simulink model "Two_Level_Inverter"  (R2016a)
settings: Solver=VariableStepAuto  StartTime=0.0  StopTime=0.3  RelTol=1e-3
libraries: powerlib x10, simulink x1
settings Model: Creator=shahinSabour  LastModifiedBy=shahin

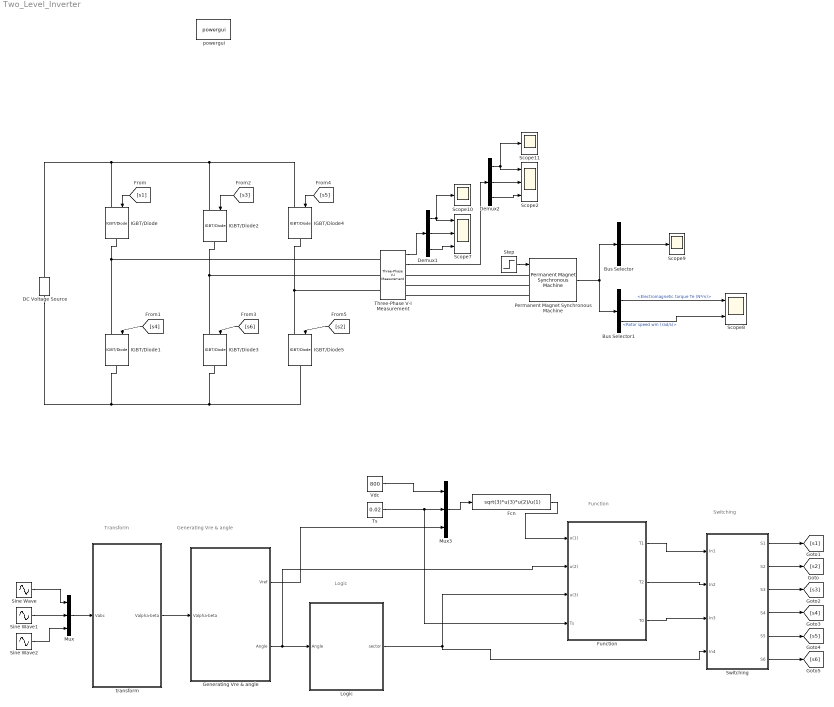
== system Two_Level_Inverter ==
  note: Transform
  note: Generating Vre & angle
  note: Logic
  note: Function
  note: Switching
  " transform" : Subsystem
  Bus Selector : BusSelector  OutputSignals=Stator current is_a (A),Stator current is_b (A),Stator current is_c (A)  OutputAsBus=on
  Bus Selector1 : BusSelector  OutputSignals=Electromagnetic torque Te (N*m),Rotor speed wm (rad/s)
  DC Voltage Source : powerlib/Electrical Sources/DC Voltage Source  Amplitude=800  Measurements=None
  Demux1 : Demux  Outputs=3
  Demux2 : Demux  Outputs=3
  Fcn : Fcn  Expr=sqrt(3)*u(3)*u(2)/u(1)
  Function : Subsystem
  Generating Vre & angle : Subsystem
  IGBT/Diode{,1..5} (6 alike) : powerlib/Power Electronics/IGBT//Diode  Ron=1e-3  Rs=1e5  Cs=inf  Measurements=off
  Logic : Subsystem
  Mux : Mux  Inputs=3
  Mux3 : Mux  Inputs=3
  Permanent Magnet Synchronous Machine : powerlib/Machines/Permanent Magnet Synchronous Machine  NbPhases=3  FluxDistribution=Sinusoidal  RotorType=Round  MechanicalLoad=Torque Tm  PresetModel="03:  2.8 Nm 300 Vdc 4250 RPM - 3.2 Nm"  ShowDetailedParameters=on  MeasurementBus=off  Resistance=1.6  Inductance=8.5e-3  dqInductances=[8.5e-3,8.5e-3]  La=0.006365  MachineConstant=Flux linkage established by magnets (V.s)  Flux=0.1852  VoltageCst=67.1831  TorqueCst=0.5556  Flat=120  Mechanical=[0.0001854 5.396e-05 2 0]  PolePairs=2  InitialConditions=[0,0, 0,0]  InitialConditions5ph=[0 0 0 0 0 0]  TsPowergui=0  TsBlock=-1  RefAngle=90 degrees behind phase A axis (modified Park)
  Scope10 : Scope
  Scope11 : Scope
  Scope2 : Scope  NumInputPorts=3
  Scope7 : Scope  NumInputPorts=3
  Scope8 : Scope  NumInputPorts=2
  Scope9 : Scope
  Sine Wave : Sin  Amplitude=800  Frequency=2*pi*50  SampleTime=0
  Sine Wave1 : Sin  Amplitude=800  Frequency=2*pi*50  Phase=2*pi/3  SampleTime=0
  Sine Wave2 : Sin  Amplitude=800  Frequency=2*pi*50  Phase=-2*pi/3  SampleTime=0
  Step : Step  Time=0.8  After=3  SampleTime=0
  "Switching " : Subsystem
  Three-Phase V-I Measurement : powerlib/Measurements/Three-Phase V-I Measurement  VoltageMeasurement=phase-to-phase  SetLabelV=off  LabelV=Vabc  Vpu=off  VpuLL=off  CurrentMeasurement=yes  SetLabelI=off  LabelI=Iabc  Ipu=off  Pbase=100e6  Vbase=500e3  OutputType=Complex  PhasorSimulation=off  PSBequivalent=0
  Ts : Constant  Value=0.02
  Vdc : Constant  Value=800
  powergui : powerlib/powergui  Priority=1  SimulationMode=Discrete  SolverType=Tustin/Backward Euler (TBE)  SampleTime=1e-7  frequency=60  SPID=off  DisableSnubberDevices=off  DisableRonSwitches=off  DisableVfSwitches=off  SwTol=0  DisplayEquations=off  Interpol=off  ExternalGateDelay=off  methode=off  Ts=10  FunctionMessages=off  echomessages=off  HookPort=off  EnableUseOfTLC=off  x0status=blocks  frequencyindice=0  Pbase=100e6  ErrMax=1e-4  Iterations=50  UnitsV=kV  UnitsW=MW  buscounter=0  RestoreLinks=warning  ResistiveCurrentMeasurement=off  Frange=[0:2:500]  Ylog=off  Xlog=on  ShowGrid=off  save=off  variable=ZData  structure=i  ZoomFFT=off  StartTime=0.2  cycles=1  DisplayStyle=1  fundamental=50  FreqAxis=on  MaxFrequency=1000  frequencyindicesteady=1  RmsSteady=1  display=off
  wires:
  Sine Wave/1 -> Mux/1
  Sine Wave1/1 -> Mux/2
  Sine Wave2/1 -> Mux/3
  Mux/1 -> " transform"/1(Vabc)
  " transform"/1(Valpha-beta) -> Generating Vre & angle/1(Valpha-beta)
  Generating Vre & angle/2(Angle) -> Function/2(u(2)), Logic/1(Angle)
  Generating Vre & angle/1(Vref) -> Mux3/3
  Ts/1 -> Function/4(Ts), Mux3/2
  Vdc/1 -> Mux3/1
  Mux3/1 -> Fcn/1
  Fcn/1 -> Function/1(u(1))
  Logic/1(sector) -> "Switching "/4(In4), Function/3(u(3))
  Permanent Magnet Synchronous Machine/1 -> Bus Selector1/1, Bus Selector/1
  Bus Selector1/1 -> Scope8/1  "<Electromagnetic torque Te (N*m)>"
  Bus Selector1/2 -> Scope8/2  "<Rotor speed wm (rad/s)>"
  Bus Selector/1 -> Scope9/1
  Step/1 -> Permanent Magnet Synchronous Machine/1
  Three-Phase V-I Measurement/1 -> Demux1/1
  Demux1/1 -> Scope10/1, Scope7/1
  Demux1/2 -> Scope7/2
  Demux1/3 -> Scope7/3
  Three-Phase V-I Measurement/2 -> Demux2/1
  Demux2/1 -> Scope2/1, Scope11/1
  Demux2/2 -> Scope2/2
  Demux2/3 -> Scope2/3
  [s5] -> IGBT/Diode4/1
  [s3] -> IGBT/Diode2/1
  [s6] -> IGBT/Diode3/1
  [s2] -> IGBT/Diode5/1
  [s4] -> IGBT/Diode1/1
  [s1] -> IGBT/Diode/1
  Function/1(T1) -> "Switching "/1(In1)
  Function/2(T2) -> "Switching "/2(In2)
  Function/3(T0) -> "Switching "/3(In3)
  "Switching "/2(S2) -> [s2]
  "Switching "/1(S1) -> [s1]
  "Switching "/3(S3) -> [s3]
  "Switching "/4(S4) -> [s4]
  "Switching "/5(S5) -> [s5]
  "Switching "/6(S6) -> [s6]
  connections:
  Permanent Magnet Synchronous Machine/LConn1 -- Three-Phase V-I Measurement/RConn1
  Permanent Magnet Synchronous Machine/LConn2 -- Three-Phase V-I Measurement/RConn2
  Permanent Magnet Synchronous Machine/LConn3 -- Three-Phase V-I Measurement/RConn3
  IGBT/Diode1/RConn1 -- DC Voltage Source/LConn1 -- IGBT/Diode3/RConn1 -- IGBT/Diode5/RConn1
  IGBT/Diode/RConn1 -- Three-Phase V-I Measurement/LConn1 -- IGBT/Diode1/LConn1
  IGBT/Diode/LConn1 -- DC Voltage Source/RConn1 -- IGBT/Diode2/LConn1 -- IGBT/Diode4/LConn1
  IGBT/Diode4/RConn1 -- Three-Phase V-I Measurement/LConn3 -- IGBT/Diode5/LConn1
  IGBT/Diode2/RConn1 -- Three-Phase V-I Measurement/LConn2 -- IGBT/Diode3/LConn1

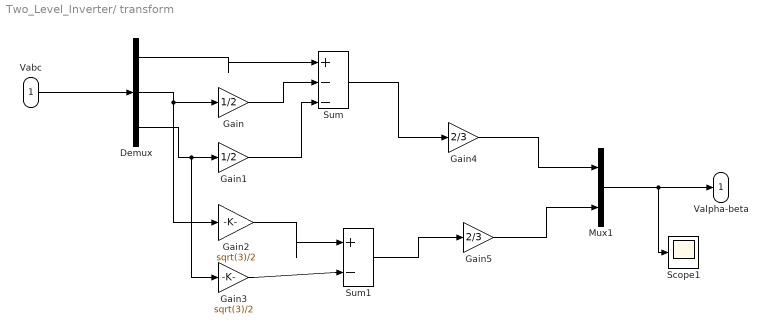
== system Two_Level_Inverter/ transform ==
  Vabc : Inport
  Demux : Demux  Outputs=3
  Gain : Gain  Gain=1/2
  Gain1 : Gain  Gain=1/2
  Gain2 : Gain  Gain=sqrt(3)/2
  Gain3 : Gain  Gain=sqrt(3)/2
  Gain4 : Gain  Gain=2/3
  Gain5 : Gain  Gain=2/3
  Mux1 : Mux  Inputs=2
  Scope1 : Scope
  Sum : Sum  Inputs=|+--
  Sum1 : Sum  Inputs=|+-
  Valpha-beta : Outport
  wires:
  Gain2/1 -> Sum1/1
  Gain5/1 -> Mux1/2
  Demux/3 -> Gain3/1, Gain1/1
  Demux/1 -> Sum/1
  Gain1/1 -> Sum/3
  Gain3/1 -> Sum1/2
  Demux/2 -> Gain2/1, Gain/1
  Mux1/1 -> Valpha-beta/1, Scope1/1
  Sum/1 -> Gain4/1
  Gain/1 -> Sum/2
  Sum1/1 -> Gain5/1
  Gain4/1 -> Mux1/1
  Vabc/1 -> Demux/1

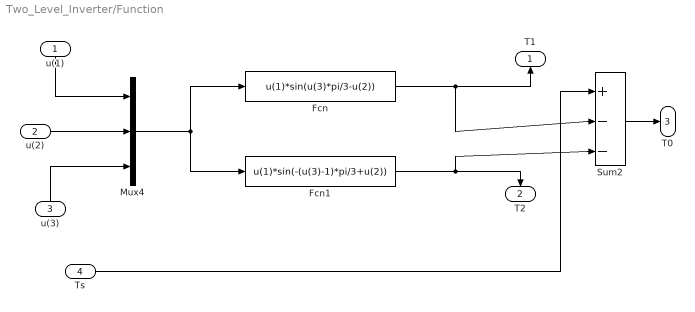
== system Two_Level_Inverter/Function ==
  u(1) : Inport
  u(2) : Inport  Port=2
  u(3) : Inport  Port=3
  Ts : Inport  Port=4
  Fcn : Fcn  Expr=u(1)*sin(u(3)*pi/3-u(2))
  Fcn1 : Fcn  Expr=u(1)*sin(-(u(3)-1)*pi/3+u(2))
  Mux4 : Mux  Inputs=3
  Sum2 : Sum  Inputs=|+--
  T1 : Outport
  T2 : Outport  Port=2
  T0 : Outport  Port=3
  wires:
  u(3)/1 -> Mux4/3
  u(2)/1 -> Mux4/2
  u(1)/1 -> Mux4/1
  Sum2/1 -> T0/1
  Fcn/1 -> Sum2/2, T1/1
  Ts/1 -> Sum2/1
  Fcn1/1 -> T2/1, Sum2/3
  Mux4/1 -> Fcn1/1, Fcn/1

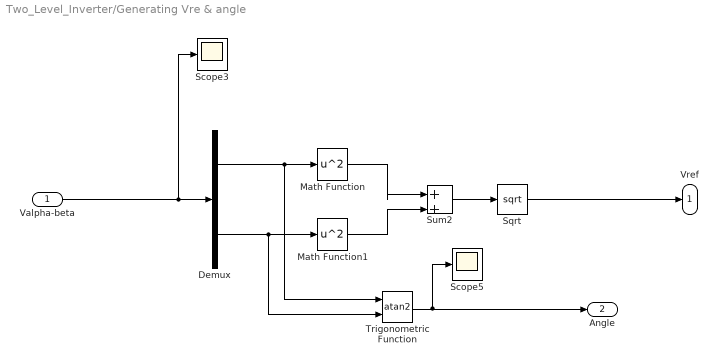
== system Two_Level_Inverter/Generating Vre & angle ==
  Valpha-beta : Inport
  Demux : Demux  Outputs=2
  Math Function : Math  Operator=square  SaturateOnIntegerOverflow=on
  Math Function1 : Math  Operator=square  SaturateOnIntegerOverflow=on
  Scope3 : Scope
  Scope5 : Scope
  Sqrt : Sqrt  SaturateOnIntegerOverflow=on
  Sum2 : Sum  Inputs=|++
  Trigonometric Function : Trigonometry  Operator=atan2
  Vref : Outport
  Angle : Outport  Port=2
  wires:
  Valpha-beta/1 -> Scope3/1, Demux/1
  Sqrt/1 -> Vref/1
  Math Function/1 -> Sum2/1
  Math Function1/1 -> Sum2/2
  Demux/2 -> Trigonometric Function/2, Math Function1/1
  Demux/1 -> Trigonometric Function/1, Math Function/1
  Sum2/1 -> Sqrt/1
  Trigonometric Function/1 -> Angle/1, Scope5/1

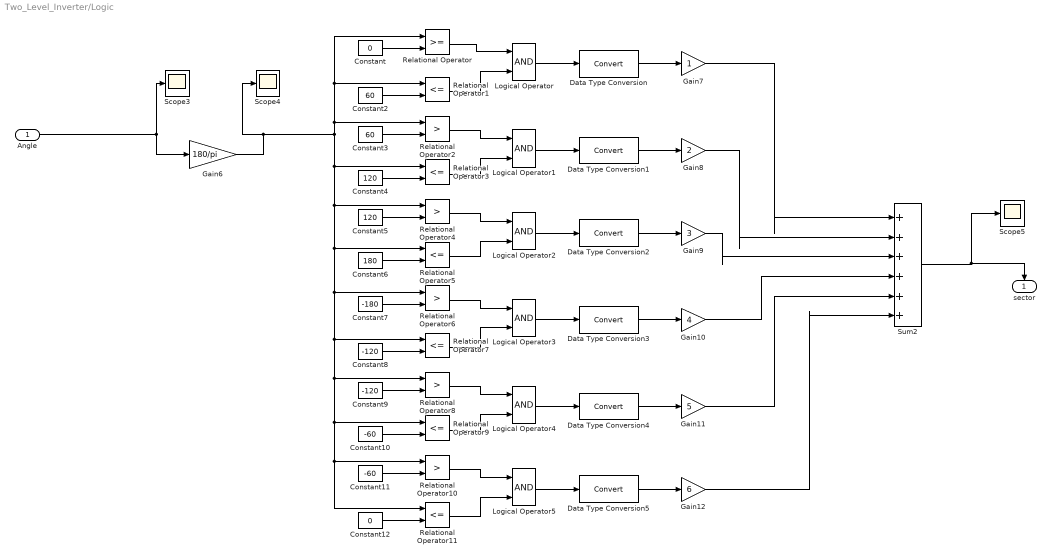
== system Two_Level_Inverter/Logic ==
  Angle : Inport
  Constant : Constant  Value=0
  Constant10 : Constant  Value=-60
  Constant11 : Constant  Value=-60
  Constant12 : Constant  Value=0
  Constant2 : Constant  Value=60
  Constant3 : Constant  Value=60
  Constant4 : Constant  Value=120
  Constant5 : Constant  Value=120
  Constant6 : Constant  Value=180
  Constant7 : Constant  Value=-180
  Constant8 : Constant  Value=-120
  Constant9 : Constant  Value=-120
  Data Type Conversion{,1..5} (6 alike) : DataTypeConversion
  Gain10 : Gain  Gain=4
  Gain11 : Gain  Gain=5
  Gain12 : Gain  Gain=6
  Gain6 : Gain  Gain=180/pi
  Gain7 : Gain
  Gain8 : Gain  Gain=2
  Gain9 : Gain  Gain=3
  Logical Operator{,1..5} (6 alike) : Logic  AllPortsSameDT=off  OutDataTypeStr=boolean
  Relational Operator : RelationalOperator  OutDataTypeStr=boolean
  Relational Operator{1,3,5,7,9,11} (6 alike) : RelationalOperator  Operator=<=  OutDataTypeStr=boolean
  Relational Operator{2,4,6,8,10} (5 alike) : RelationalOperator  Operator=>  OutDataTypeStr=boolean
  Scope3 : Scope
  Scope4 : Scope
  Scope5 : Scope
  Sum2 : Sum  Inputs=|++++++
  sector : Outport
  wires:
  Relational Operator3/1 -> Logical Operator1/2
  Data Type Conversion4/1 -> Gain11/1
  Logical Operator4/1 -> Data Type Conversion4/1
  Constant4/1 -> Relational Operator3/2
  Gain12/1 -> Sum2/6
  Constant11/1 -> Relational Operator10/2
  Constant10/1 -> Relational Operator9/2
  Constant8/1 -> Relational Operator7/2
  Constant9/1 -> Relational Operator8/2
  Relational Operator4/1 -> Logical Operator2/1
  Relational Operator7/1 -> Logical Operator3/2
  Data Type Conversion5/1 -> Gain12/1
  Logical Operator5/1 -> Data Type Conversion5/1
  Logical Operator1/1 -> Data Type Conversion1/1
  Data Type Conversion1/1 -> Gain8/1
  Gain8/1 -> Sum2/2
  Constant7/1 -> Relational Operator6/2
  Logical Operator3/1 -> Data Type Conversion3/1
  Data Type Conversion2/1 -> Gain9/1
  Logical Operator2/1 -> Data Type Conversion2/1
  Logical Operator/1 -> Data Type Conversion/1
  Gain7/1 -> Sum2/1
  Gain10/1 -> Sum2/4
  Relational Operator1/1 -> Logical Operator/2
  Relational Operator5/1 -> Logical Operator2/2
  Constant3/1 -> Relational Operator2/2
  Constant5/1 -> Relational Operator4/2
  Constant12/1 -> Relational Operator11/2
  Relational Operator/1 -> Logical Operator/1
  Constant2/1 -> Relational Operator1/2
  Relational Operator11/1 -> Logical Operator5/2
  Relational Operator9/1 -> Logical Operator4/2
  Data Type Conversion/1 -> Gain7/1
  Constant6/1 -> Relational Operator5/2
  Relational Operator6/1 -> Logical Operator3/1
  Gain9/1 -> Sum2/3
  Sum2/1 -> sector/1, Scope5/1
  Gain11/1 -> Sum2/5
  Data Type Conversion3/1 -> Gain10/1
  Constant/1 -> Relational Operator/2
  Relational Operator8/1 -> Logical Operator4/1
  Gain6/1 -> Scope4/1, Relational Operator3/1, Relational Operator4/1, Relational Operator5/1, Relational Operator6/1, Relational Operator7/1, Relational Operator8/1, Relational Operator9/1, Relational Operator10/1, Relational Operator11/1, Relational Operator2/1, Relational Operator1/1, Relational Operator/1
  Relational Operator2/1 -> Logical Operator1/1
  Angle/1 -> Scope3/1, Gain6/1
  Relational Operator10/1 -> Logical Operator5/1

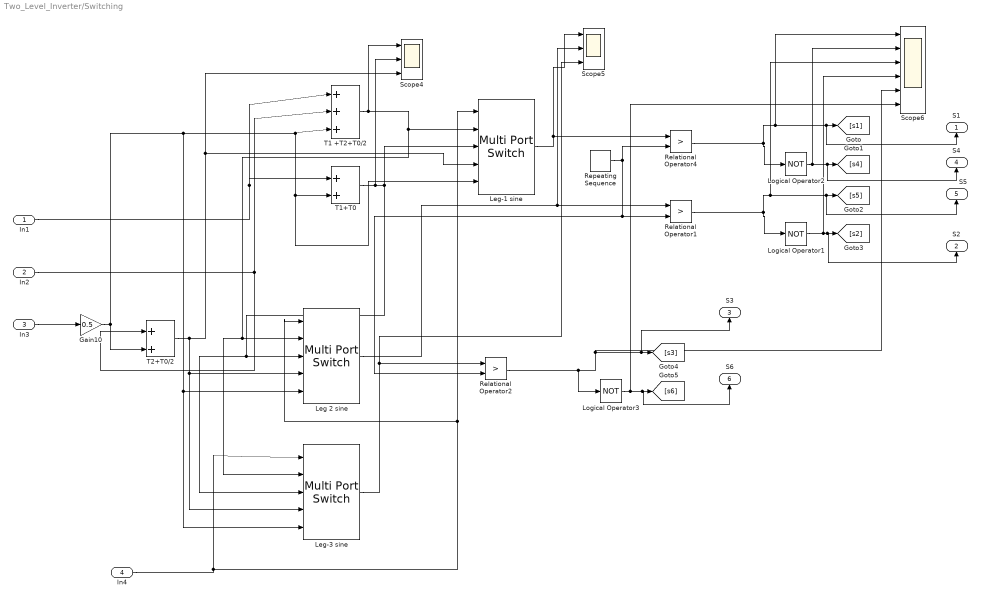
== system Two_Level_Inverter/Switching  ==
  In1 : Inport
  In2 : Inport  Port=2
  In3 : Inport  Port=3
  In4 : Inport  Port=4
  Gain10 : Gain  Gain=0.5
  Leg 2 sine : MultiPortSwitch  DataPortOrder=Specify indices  DataPortIndices={[2,3],4,1,[5,6]}  DiagnosticForDefault=None
  Leg-1 sine : MultiPortSwitch  DataPortOrder=Specify indices  DataPortIndices={[1,6],2,5,[3,4]}  DiagnosticForDefault=None
  Leg-3 sine : MultiPortSwitch  DataPortOrder=Specify indices  DataPortIndices={[4,5],6,3,[1,2]}  DiagnosticForDefault=None
  Logical Operator1 : Logic  Operator=NOT  AllPortsSameDT=off  OutDataTypeStr=boolean
  Logical Operator2 : Logic  Operator=NOT  AllPortsSameDT=off  OutDataTypeStr=boolean
  Logical Operator3 : Logic  Operator=NOT  AllPortsSameDT=off  OutDataTypeStr=boolean
  Relational Operator1 : RelationalOperator  Operator=>  OutDataTypeStr=boolean
  Relational Operator2 : RelationalOperator  Operator=>  OutDataTypeStr=boolean
  Relational Operator4 : RelationalOperator  Operator=>  OutDataTypeStr=boolean
  Repeating Sequence : simulink/Sources/Repeating Sequence  rep_seq_t=[0 1]*[1/2000]  rep_seq_y=[0 0.02]
  Scope4 : Scope  NumInputPorts=3
  Scope5 : Scope  NumInputPorts=3
  Scope6 : Scope  NumInputPorts=6
  T1 +T2+T0/2 : Sum  Inputs=|+++
  T1+T0 : Sum  Inputs=|++
  T2+T0/2 : Sum  Inputs=|++
  S1 : Outport
  S2 : Outport  Port=2
  S3 : Outport  Port=3
  S4 : Outport  Port=4
  S5 : Outport  Port=5
  S6 : Outport  Port=6
  wires:
  In4/1 -> Leg-3 sine/1, Leg-1 sine/1, Leg 2 sine/1
  In3/1 -> Gain10/1
  Gain10/1 -> Leg-1 sine/5, T1+T0/2, T1 +T2+T0/2/3, Leg-3 sine/5, Leg 2 sine/5, T2+T0/2/2
  In2/1 -> T1 +T2+T0/2/2, T2+T0/2/1
  In1/1 -> T1 +T2+T0/2/1, T1+T0/1
  T1 +T2+T0/2/1 -> Scope4/1, Leg-3 sine/2, Leg 2 sine/2, Leg-1 sine/2
  Repeating Sequence/1 -> Relational Operator1/2, Relational Operator2/2, Relational Operator4/2
  Leg-1 sine/1 -> Scope5/1, Relational Operator4/1
  T1+T0/1 -> Leg-1 sine/3, Leg-3 sine/3, Leg 2 sine/3, Scope4/2
  Leg 2 sine/1 -> Relational Operator1/1, Scope5/2
  Leg-3 sine/1 -> Relational Operator2/1, Scope5/3
  Relational Operator4/1 -> Logical Operator2/1, Scope6/1, S1/1, [s1]
  T2+T0/2/1 -> Scope4/3, Leg-1 sine/4, Leg-3 sine/4, Leg 2 sine/4
  Logical Operator2/1 -> Scope6/2, S4/1, [s4]
  Relational Operator2/1 -> Logical Operator3/1, Scope6/5, S3/1, [s3]
  Logical Operator1/1 -> Scope6/4, S2/1, [s2]
  Relational Operator1/1 -> Logical Operator1/1, Scope6/3, S5/1, [s5]
  Logical Operator3/1 -> Scope6/6, S6/1, [s6]
